simulink model "SST_5"  (R2022b)
settings: Solver=VariableStepAuto  StartTime=0.0  StopTime=1.0  RelTol=1e-3
libraries: spsSeriesRLCBranchLib x13, spsIGBTDiodeLib x10, spsMosfetLib x6, slpidlib x5, spsCurrentMeasurementLib x4, spsDiodeLib x4, spsThreePhaseVIMeasurementLib x3, spsAlphaBetaZerotodq0Lib x2, spsThreePhaseSeriesRLCBranchLib x2, spsVoltageMeasurementLib x2, spsLinearTransformerLib x1, spsGroundLib x1
settings Model: Creator=DR. AGBARAJI  LastModifiedBy=DR. AGBARAJI

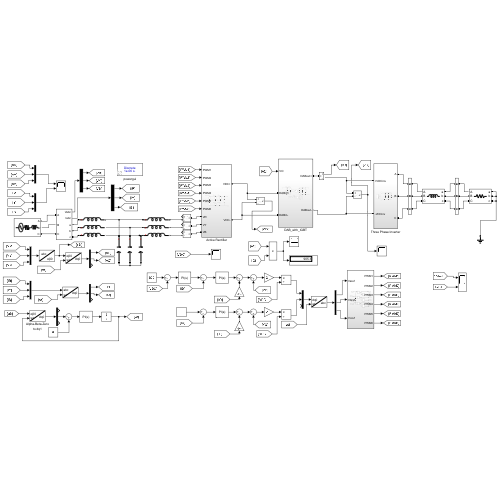
[thumbnail: Simulink's stored preview of the top-level diagram]
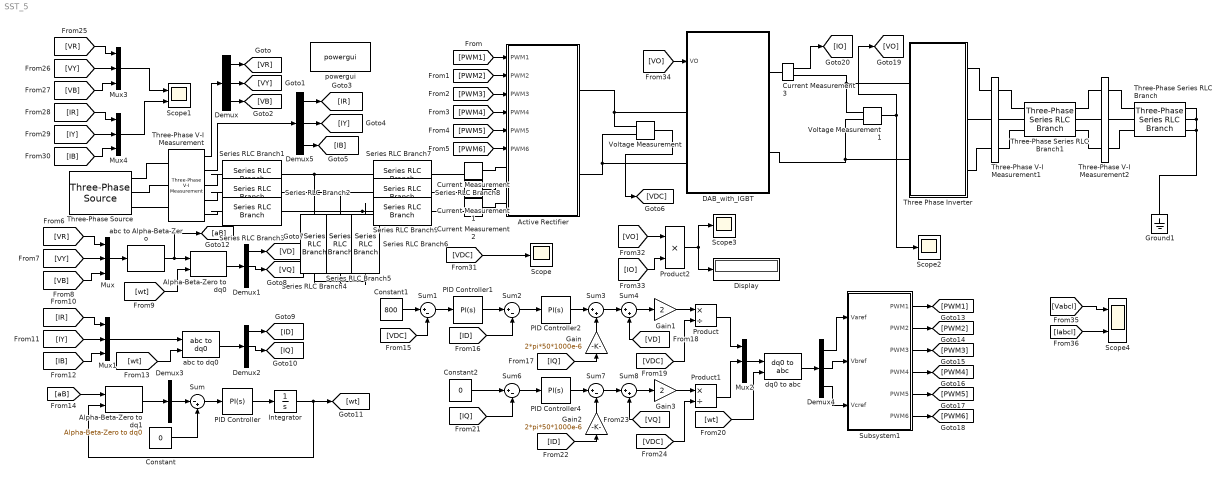
== system SST_5 ==
  Active Rectifier : Subsystem
  Alpha-Beta-Zero to dq0 : spsAlphaBetaZerotodq0Lib/Alpha-Beta-Zero to dq0  Alignment=90 degrees behind phase A axis
  Alpha-Beta-Zero to dq1 : spsAlphaBetaZerotodq0Lib/Alpha-Beta-Zero to dq0  Alignment=90 degrees behind phase A axis
  Constant : Constant  Value=0
  Constant1 : Constant  Value=800
  Constant2 : Constant  Value=0
  Current Measurement{,1..3} (4 alike) : spsCurrentMeasurementLib/Current Measurement  PhasorSimulation=off  OutputType=Complex  PSBequivalent=0
  DAB_with_IGBT : Subsystem
  Demux{,1..5} (6 alike) : Demux  Outputs=3
  Display : Display
  Gain : Gain  Gain=2*pi*50*1000e-6
  Gain1 : Gain  Gain=2
  Gain2 : Gain  Gain=2*pi*50*1000e-6
  Gain3 : Gain  Gain=2
  Ground1 : spsGroundLib/Ground  LConnTagsString=a
  Integrator : Integrator
  Mux{,1..4} (5 alike) : Mux  Inputs=3
  PID Controller : slpidlib/PID Controller  Controller=PI  Form=Parallel  TimeDomain=Continuous-time  UseExternalTs=off  SampleTime=-1  IntegratorMethod=Forward Euler  FilterMethod=Forward Euler  ControllerParametersSource=internal  P=10  I=50000  UseKiTs=off  D=0  N=100  UseFilter=on  TunerSelectOption=Transfer Function Based (PID Tuner App)  InitialConditionSource=internal  InitialConditionForIntegrator=0  InitialConditionForFilter=0  DifferentiatorICPrevScaledInput=0  ExternalReset=none  TrackingMode=off  Kt=1  LimitOutput=off  SatLimitsSource=internal  UpperSaturationLimit=inf  LowerSaturationLimit=-inf  LinearizeAsGain=on  AntiWindupMode=none  Kb=1  LimitIntegrator=off  UpperIntegratorSaturationLimit=inf  LowerIntegratorSaturationLimit=-inf  POutMin=[]  POutMax=[]  IOutMin=[]  IOutMax=[]  DOutMin=[]  DOutMax=[]  NOutMin=[]  NOutMax=[]  SumOutMin=[]  SumOutMax=[]  SaturationOutMin=[]  SaturationOutMax=[]  PParamMin=[]  PParamMax=[]  IParamMin=[]  IParamMax=[]  DParamMin=[]  DParamMax=[]  NParamMin=[]  NParamMax=[]  KbParamMin=[]  KbParamMax=[]  KtParamMin=[]  KtParamMax=[]  KbOutMin=[]  KbOutMax=[]  KtOutMin=[]  KtOutMax=[]  IntegratorOutMin=[]  IntegratorOutMax=[]  FilterOutMin=[]  FilterOutMax=[]  SumI1OutMin=[]  SumI1OutMax=[]  SumI2OutMin=[]  SumI2OutMax=[]  SumI3OutMin=[]  SumI3OutMax=[]  SumI4OutMin=[]  SumI4OutMax=[]  SumDOutMin=[]  SumDOutMax=[]  DifferentiatorOutMin=[]  DifferentiatorOutMax=[]  FilterDiffOutCoefMin=[]  FilterDiffOutCoefMax=[]  ReciprocalOutMin=[]  ReciprocalOutMax=[]  SumDenOutMin=[]  SumDenOutMax=[]  SumNumOutMin=[]  SumNumOutMax=[]  DivideOutMin=[]  DivideOutMax=[]  UdiffTsProdOutMin=[]  UdiffTsProdOutMax=[]  NTsProdOutMin=[]  NTsProdOutMax=[]  UintegralTsProdOutMin=[]  UintegralTsProdOutMax=[]  UngainTsProdOutMin=[]  UngainTsProdOutMax=[]  ClampingZeroOutDataTypeStr=Inherit: Inherit via back propagation  ClampingZeroOutMin=[]  ClampingZeroOutMax=[]  FilterDenConstantOutDataTypeStr=Inherit: Inherit via back propagation  FilterDenConstantOutMin=[]  FilterDenConstantOutMax=[]  PCopyOutDataTypeStr=Inherit: Inherit via back propagation  PCopyOutMin=[]  PCopyOutMax=[]  NCopyOutDataTypeStr=Inherit: Inherit via back propagation  NCopyOutMin=[]  NCopyOutMax=[]  IntegratorContinuousStateAttributes=''  IntegratorStateMustResolveToSignalObject=off  IntegratorRTWStateStorageClass=Auto  FilterContinuousStateAttributes=''  FilterStateMustResolveToSignalObject=off  FilterRTWStateStorageClass=Auto  ParallelPVariant=InternalParameters  IdealPVariant=Disabled  IVariant=InternalParameters  DVariant=Disabled  IntegratorVariant=Continuous  SatVariant=Disabled  AWVariant=Passthrough  PCopyVariant=Disabled  TRVariant=Disabled  FdbkBlocksVariant=Forward  IdealPFdbkVariant=Disabled  SatFdbkVariant=Disabled  DerivativeFilterVariant=Disabled  NVariant=Disabled  NCopyVariant=Disabled_SignalSpec  FilterICVariant=Disabled  IntegratorICVariant=InternalICs  ExternalResetVariant=Disabled  TRSumVariant=Passthrough  SumFdbkVariant=Disabled  SumVariant=Sum_PI  TsampFilterVariant=InternalTs  TsampNgainVariant=Passthrough  TsampIntegralVariant=Passthrough  ExternalSaturationOutDataTypeStr=Inherit: Same as second input
  PID Controller1 : slpidlib/PID Controller  Controller=PI  Form=Parallel  TimeDomain=Continuous-time  UseExternalTs=off  SampleTime=-1  IntegratorMethod=Forward Euler  FilterMethod=Forward Euler  ControllerParametersSource=internal  P=0.5  I=200  UseKiTs=off  D=0  N=100  UseFilter=on  TunerSelectOption=Transfer Function Based (PID Tuner App)  InitialConditionSource=internal  InitialConditionForIntegrator=0  InitialConditionForFilter=0  DifferentiatorICPrevScaledInput=0  ExternalReset=none  TrackingMode=off  Kt=1  LimitOutput=off  SatLimitsSource=internal  UpperSaturationLimit=inf  LowerSaturationLimit=-inf  LinearizeAsGain=on  AntiWindupMode=none  Kb=1  LimitIntegrator=off  UpperIntegratorSaturationLimit=inf  LowerIntegratorSaturationLimit=-inf  POutMin=[]  POutMax=[]  IOutMin=[]  IOutMax=[]  DOutMin=[]  DOutMax=[]  NOutMin=[]  NOutMax=[]  SumOutMin=[]  SumOutMax=[]  SaturationOutMin=[]  SaturationOutMax=[]  PParamMin=[]  PParamMax=[]  IParamMin=[]  IParamMax=[]  DParamMin=[]  DParamMax=[]  NParamMin=[]  NParamMax=[]  KbParamMin=[]  KbParamMax=[]  KtParamMin=[]  KtParamMax=[]  KbOutMin=[]  KbOutMax=[]  KtOutMin=[]  KtOutMax=[]  IntegratorOutMin=[]  IntegratorOutMax=[]  FilterOutMin=[]  FilterOutMax=[]  SumI1OutMin=[]  SumI1OutMax=[]  SumI2OutMin=[]  SumI2OutMax=[]  SumI3OutMin=[]  SumI3OutMax=[]  SumI4OutMin=[]  SumI4OutMax=[]  SumDOutMin=[]  SumDOutMax=[]  DifferentiatorOutMin=[]  DifferentiatorOutMax=[]  FilterDiffOutCoefMin=[]  FilterDiffOutCoefMax=[]  ReciprocalOutMin=[]  ReciprocalOutMax=[]  SumDenOutMin=[]  SumDenOutMax=[]  SumNumOutMin=[]  SumNumOutMax=[]  DivideOutMin=[]  DivideOutMax=[]  UdiffTsProdOutMin=[]  UdiffTsProdOutMax=[]  NTsProdOutMin=[]  NTsProdOutMax=[]  UintegralTsProdOutMin=[]  UintegralTsProdOutMax=[]  UngainTsProdOutMin=[]  UngainTsProdOutMax=[]  ClampingZeroOutDataTypeStr=Inherit: Inherit via back propagation  ClampingZeroOutMin=[]  ClampingZeroOutMax=[]  FilterDenConstantOutDataTypeStr=Inherit: Inherit via back propagation  FilterDenConstantOutMin=[]  FilterDenConstantOutMax=[]  PCopyOutDataTypeStr=Inherit: Inherit via back propagation  PCopyOutMin=[]  PCopyOutMax=[]  NCopyOutDataTypeStr=Inherit: Inherit via back propagation  NCopyOutMin=[]  NCopyOutMax=[]  IntegratorContinuousStateAttributes=''  IntegratorStateMustResolveToSignalObject=off  IntegratorRTWStateStorageClass=Auto  FilterContinuousStateAttributes=''  FilterStateMustResolveToSignalObject=off  FilterRTWStateStorageClass=Auto  ParallelPVariant=InternalParameters  IdealPVariant=Disabled  IVariant=InternalParameters  DVariant=Disabled  IntegratorVariant=Continuous  SatVariant=Disabled  AWVariant=Passthrough  PCopyVariant=Disabled  TRVariant=Disabled  FdbkBlocksVariant=Forward  IdealPFdbkVariant=Disabled  SatFdbkVariant=Disabled  DerivativeFilterVariant=Disabled  NVariant=Disabled  NCopyVariant=Disabled_SignalSpec  FilterICVariant=Disabled  IntegratorICVariant=InternalICs  ExternalResetVariant=Disabled  TRSumVariant=Passthrough  SumFdbkVariant=Disabled  SumVariant=Sum_PI  TsampFilterVariant=InternalTs  TsampNgainVariant=Passthrough  TsampIntegralVariant=Passthrough  ExternalSaturationOutDataTypeStr=Inherit: Same as second input
  PID Controller2 : slpidlib/PID Controller  Controller=PI  Form=Parallel  TimeDomain=Continuous-time  UseExternalTs=off  SampleTime=-1  IntegratorMethod=Forward Euler  FilterMethod=Forward Euler  ControllerParametersSource=internal  P=25  I=500  UseKiTs=off  D=0  N=100  UseFilter=on  TunerSelectOption=Transfer Function Based (PID Tuner App)  InitialConditionSource=internal  InitialConditionForIntegrator=0  InitialConditionForFilter=0  DifferentiatorICPrevScaledInput=0  ExternalReset=none  TrackingMode=off  Kt=1  LimitOutput=off  SatLimitsSource=internal  UpperSaturationLimit=inf  LowerSaturationLimit=-inf  LinearizeAsGain=on  AntiWindupMode=none  Kb=1  LimitIntegrator=off  UpperIntegratorSaturationLimit=inf  LowerIntegratorSaturationLimit=-inf  POutMin=[]  POutMax=[]  IOutMin=[]  IOutMax=[]  DOutMin=[]  DOutMax=[]  NOutMin=[]  NOutMax=[]  SumOutMin=[]  SumOutMax=[]  SaturationOutMin=[]  SaturationOutMax=[]  PParamMin=[]  PParamMax=[]  IParamMin=[]  IParamMax=[]  DParamMin=[]  DParamMax=[]  NParamMin=[]  NParamMax=[]  KbParamMin=[]  KbParamMax=[]  KtParamMin=[]  KtParamMax=[]  KbOutMin=[]  KbOutMax=[]  KtOutMin=[]  KtOutMax=[]  IntegratorOutMin=[]  IntegratorOutMax=[]  FilterOutMin=[]  FilterOutMax=[]  SumI1OutMin=[]  SumI1OutMax=[]  SumI2OutMin=[]  SumI2OutMax=[]  SumI3OutMin=[]  SumI3OutMax=[]  SumI4OutMin=[]  SumI4OutMax=[]  SumDOutMin=[]  SumDOutMax=[]  DifferentiatorOutMin=[]  DifferentiatorOutMax=[]  FilterDiffOutCoefMin=[]  FilterDiffOutCoefMax=[]  ReciprocalOutMin=[]  ReciprocalOutMax=[]  SumDenOutMin=[]  SumDenOutMax=[]  SumNumOutMin=[]  SumNumOutMax=[]  DivideOutMin=[]  DivideOutMax=[]  UdiffTsProdOutMin=[]  UdiffTsProdOutMax=[]  NTsProdOutMin=[]  NTsProdOutMax=[]  UintegralTsProdOutMin=[]  UintegralTsProdOutMax=[]  UngainTsProdOutMin=[]  UngainTsProdOutMax=[]  ClampingZeroOutDataTypeStr=Inherit: Inherit via back propagation  ClampingZeroOutMin=[]  ClampingZeroOutMax=[]  FilterDenConstantOutDataTypeStr=Inherit: Inherit via back propagation  FilterDenConstantOutMin=[]  FilterDenConstantOutMax=[]  PCopyOutDataTypeStr=Inherit: Inherit via back propagation  PCopyOutMin=[]  PCopyOutMax=[]  NCopyOutDataTypeStr=Inherit: Inherit via back propagation  NCopyOutMin=[]  NCopyOutMax=[]  IntegratorContinuousStateAttributes=''  IntegratorStateMustResolveToSignalObject=off  IntegratorRTWStateStorageClass=Auto  FilterContinuousStateAttributes=''  FilterStateMustResolveToSignalObject=off  FilterRTWStateStorageClass=Auto  ParallelPVariant=InternalParameters  IdealPVariant=Disabled  IVariant=InternalParameters  DVariant=Disabled  IntegratorVariant=Continuous  SatVariant=Disabled  AWVariant=Passthrough  PCopyVariant=Disabled  TRVariant=Disabled  FdbkBlocksVariant=Forward  IdealPFdbkVariant=Disabled  SatFdbkVariant=Disabled  DerivativeFilterVariant=Disabled  NVariant=Disabled  NCopyVariant=Disabled_SignalSpec  FilterICVariant=Disabled  IntegratorICVariant=InternalICs  ExternalResetVariant=Disabled  TRSumVariant=Passthrough  SumFdbkVariant=Disabled  SumVariant=Sum_PI  TsampFilterVariant=InternalTs  TsampNgainVariant=Passthrough  TsampIntegralVariant=Passthrough  ExternalSaturationOutDataTypeStr=Inherit: Same as second input
  PID Controller4 : slpidlib/PID Controller  Controller=PI  Form=Parallel  TimeDomain=Continuous-time  UseExternalTs=off  SampleTime=-1  IntegratorMethod=Forward Euler  FilterMethod=Forward Euler  ControllerParametersSource=internal  P=25  I=500  UseKiTs=off  D=0  N=100  UseFilter=on  TunerSelectOption=Transfer Function Based (PID Tuner App)  InitialConditionSource=internal  InitialConditionForIntegrator=0  InitialConditionForFilter=0  DifferentiatorICPrevScaledInput=0  ExternalReset=none  TrackingMode=off  Kt=1  LimitOutput=off  SatLimitsSource=internal  UpperSaturationLimit=inf  LowerSaturationLimit=-inf  LinearizeAsGain=on  AntiWindupMode=none  Kb=1  LimitIntegrator=off  UpperIntegratorSaturationLimit=inf  LowerIntegratorSaturationLimit=-inf  POutMin=[]  POutMax=[]  IOutMin=[]  IOutMax=[]  DOutMin=[]  DOutMax=[]  NOutMin=[]  NOutMax=[]  SumOutMin=[]  SumOutMax=[]  SaturationOutMin=[]  SaturationOutMax=[]  PParamMin=[]  PParamMax=[]  IParamMin=[]  IParamMax=[]  DParamMin=[]  DParamMax=[]  NParamMin=[]  NParamMax=[]  KbParamMin=[]  KbParamMax=[]  KtParamMin=[]  KtParamMax=[]  KbOutMin=[]  KbOutMax=[]  KtOutMin=[]  KtOutMax=[]  IntegratorOutMin=[]  IntegratorOutMax=[]  FilterOutMin=[]  FilterOutMax=[]  SumI1OutMin=[]  SumI1OutMax=[]  SumI2OutMin=[]  SumI2OutMax=[]  SumI3OutMin=[]  SumI3OutMax=[]  SumI4OutMin=[]  SumI4OutMax=[]  SumDOutMin=[]  SumDOutMax=[]  DifferentiatorOutMin=[]  DifferentiatorOutMax=[]  FilterDiffOutCoefMin=[]  FilterDiffOutCoefMax=[]  ReciprocalOutMin=[]  ReciprocalOutMax=[]  SumDenOutMin=[]  SumDenOutMax=[]  SumNumOutMin=[]  SumNumOutMax=[]  DivideOutMin=[]  DivideOutMax=[]  UdiffTsProdOutMin=[]  UdiffTsProdOutMax=[]  NTsProdOutMin=[]  NTsProdOutMax=[]  UintegralTsProdOutMin=[]  UintegralTsProdOutMax=[]  UngainTsProdOutMin=[]  UngainTsProdOutMax=[]  ClampingZeroOutDataTypeStr=Inherit: Inherit via back propagation  ClampingZeroOutMin=[]  ClampingZeroOutMax=[]  FilterDenConstantOutDataTypeStr=Inherit: Inherit via back propagation  FilterDenConstantOutMin=[]  FilterDenConstantOutMax=[]  PCopyOutDataTypeStr=Inherit: Inherit via back propagation  PCopyOutMin=[]  PCopyOutMax=[]  NCopyOutDataTypeStr=Inherit: Inherit via back propagation  NCopyOutMin=[]  NCopyOutMax=[]  IntegratorContinuousStateAttributes=''  IntegratorStateMustResolveToSignalObject=off  IntegratorRTWStateStorageClass=Auto  FilterContinuousStateAttributes=''  FilterStateMustResolveToSignalObject=off  FilterRTWStateStorageClass=Auto  ParallelPVariant=InternalParameters  IdealPVariant=Disabled  IVariant=InternalParameters  DVariant=Disabled  IntegratorVariant=Continuous  SatVariant=Disabled  AWVariant=Passthrough  PCopyVariant=Disabled  TRVariant=Disabled  FdbkBlocksVariant=Forward  IdealPFdbkVariant=Disabled  SatFdbkVariant=Disabled  DerivativeFilterVariant=Disabled  NVariant=Disabled  NCopyVariant=Disabled_SignalSpec  FilterICVariant=Disabled  IntegratorICVariant=InternalICs  ExternalResetVariant=Disabled  TRSumVariant=Passthrough  SumFdbkVariant=Disabled  SumVariant=Sum_PI  TsampFilterVariant=InternalTs  TsampNgainVariant=Passthrough  TsampIntegralVariant=Passthrough  ExternalSaturationOutDataTypeStr=Inherit: Same as second input
  Product : Product  Inputs=*/
  Product1 : Product  Inputs=*/
  Product2 : Product
  Scope : Scope
  Scope1 : Scope  NumInputPorts=2
  Scope2 : Scope
  Scope3 : Scope
  Scope4 : Scope  NumInputPorts=2
  Series RLC Branch{1..3,7..9} (6 alike) : spsSeriesRLCBranchLib/Series RLC Branch  LConnTagsString=__new0  RConnTagsString=__new0  BranchType=L  Resistance=1  Inductance=500e-6  SetiL0=off  InitialCurrent=0  Capacitance=1e-6  Setx0=off  InitialVoltage=0  Measurements=None
  Series RLC Branch4 : spsSeriesRLCBranchLib/Series RLC Branch  LConnTagsString=__new0  RConnTagsString=__new0  BranchType=C  Resistance=1  Inductance=1e-3  SetiL0=off  InitialCurrent=0  Capacitance=100e-6  Setx0=off  InitialVoltage=0  Measurements=None
  Series RLC Branch5 : spsSeriesRLCBranchLib/Series RLC Branch  LConnTagsString=__new0  RConnTagsString=__new0  BranchType=C  Resistance=1  Inductance=1e-3  SetiL0=off  InitialCurrent=0  Capacitance=100e-6  Setx0=off  InitialVoltage=0  Measurements=None
  Series RLC Branch6 : spsSeriesRLCBranchLib/Series RLC Branch  LConnTagsString=__new0  RConnTagsString=__new0  BranchType=C  Resistance=1  Inductance=1e-3  SetiL0=off  InitialCurrent=0  Capacitance=100e-6  Setx0=off  InitialVoltage=0  Measurements=None
  Subsystem1 : Subsystem
  Sum : Sum  Inputs=|-+
  Sum{1..2,6..7} (4 alike) : Sum  Inputs=|+-
  Sum3 : Sum  Inputs=|++
  Sum4 : Sum  Inputs=|++
  Sum8 : Sum  Inputs=|++
  Three Phase Inverter : Subsystem
  Three-Phase Series RLC Branch : spsThreePhaseSeriesRLCBranchLib/Three-Phase Series RLC Branch  LConnTagsString=A|B|C  RConnTagsString=A|B|C  BranchType=R  Resistance=80  Inductance=1e-3  Capacitance=1e-6  Measurements=None
  Three-Phase Series RLC Branch1 : spsThreePhaseSeriesRLCBranchLib/Three-Phase Series RLC Branch  LConnTagsString=A|B|C  RConnTagsString=A|B|C  BranchType=L  Resistance=1  Inductance=9e-3  Capacitance=1e-6  Measurements=None
  Three-Phase V-I Measurement : spsThreePhaseVIMeasurementLib/Three-Phase V-I Measurement  VoltageMeasurement=phase-to-phase  SetLabelV=off  LabelV=Vabc  Vpu=off  VpuLL=off  CurrentMeasurement=yes  SetLabelI=off  LabelI=Iabc  Ipu=off  Pbase=100e6  Vbase=500e3  OutputType=Complex  PhasorSimulation=off  PSBequivalent=0
  Three-Phase V-I Measurement1 : spsThreePhaseVIMeasurementLib/Three-Phase V-I Measurement  VoltageMeasurement=phase-to-ground  SetLabelV=on  LabelV=Vabc  Vpu=off  VpuLL=off  CurrentMeasurement=yes  SetLabelI=on  LabelI=Iabc  Ipu=off  Pbase=100e6  Vbase=500e3  OutputType=Complex  PhasorSimulation=off  PSBequivalent=0
  Three-Phase V-I Measurement2 : spsThreePhaseVIMeasurementLib/Three-Phase V-I Measurement  VoltageMeasurement=phase-to-ground  SetLabelV=on  LabelV=Vabcl  Vpu=off  VpuLL=off  CurrentMeasurement=yes  SetLabelI=on  LabelI=Iabcl  Ipu=off  Pbase=100e6  Vbase=500e3  OutputType=Complex  PhasorSimulation=off  PSBequivalent=0
  Three-Phase Source : spsThreePhaseSourceLib/Three-Phase Source  InternalConnection=Y  VoltagePhases=off  Voltage=415  PhaseAngle=0  Voltage_phases=[25e3 25e3 25e3]/sqrt(3)  PhaseAngles_phases=[0 -120 +120]  Frequency=50  NonIdealSource=on  SpecifyImpedance=off  Resistance=0.8929e-3  Inductance=16.58e-6  ShortCircuitLevel=100e6  BaseVoltage=415  XRratio=7  BusType=swing  Pref=10e3  Qref=0  Prefabc=[10e3, 10e3, 10e3]  Qrefabc=[0, 0, 0]  Qmin=-inf  Qmax=inf
  Voltage Measurement : spsVoltageMeasurementLib/Voltage Measurement  PhasorSimulation=off  OutputType=Complex  PSBequivalent=0
  Voltage Measurement1 : spsVoltageMeasurementLib/Voltage Measurement  PhasorSimulation=off  OutputType=Complex  PSBequivalent=0
  abc to Alpha-Beta-Zero : spsabctoAlphaBetaZeroLib/abc to Alpha-Beta-Zero
  abc to dq0 : spsabctodq0Lib/abc to dq0  Alignment=90 degrees behind phase A axis
  dq0 to abc : spsdq0toabcLib/dq0 to abc  Alignment=90 degrees behind phase A axis
  powergui : sps_lib/powergui  Priority=1  SimulationMode=Discrete  SampleTime=1e-6  frequency=60  Iterations=50  frequencyindice=50  Pbase=100e6  ErrMax=1e-4  UnitsV=kV  UnitsW=MW  buscounter=0  FunctionMessages=off  echomessages=off  EnableUseOfTLC=off  CurrentSourceSwitches=off  DisableSnubberDevices=off  DisableRonSwitches=off  DisableVfSwitches=off  DisplayEquations=off  AutomaticDiscreteSolvers=off  SolverType=Tustin/Backward Euler (TBE)  Interpol=off  ExternalGateDelay=off  methode=off  Ts=100  x0status=blocks  SPID=on  SwTol=0  HookPort=off  NonlinearTolerance=1e-4  nMaxIteration=100  ContinueOnMaxIteration=off  RestoreLinks=warning  ResistiveCurrentMeasurement=off  Frange=[0:2:500]  Ylog=off  Xlog=on  ShowGrid=off  save=off  variable=ZData  structure=0  ZoomFFT=off  StartTime=0.0  cycles=1  DisplayStyle=1  fundamental=60  FreqAxis=off  MaxFrequency=1000  frequencyindicesteady=1  RmsSteady=1  display=off
  wires:
  Demux3/2 -> Sum/1
  [wt] -> abc to dq0/2
  Demux1/2 -> [VQ]
  [wt] -> Alpha-Beta-Zero to dq0/2
  Demux1/1 -> [VD]
  Mux/1 -> abc to Alpha-Beta-Zero/1
  [VY] -> Mux/2
  [VR] -> Mux/1
  abc to Alpha-Beta-Zero/1 -> [aB], Alpha-Beta-Zero to dq0/1
  [IR] -> Mux1/1
  Demux2/2 -> [IQ]
  [PWM5] -> Active Rectifier/5(PWM5)
  [PWM6] -> Active Rectifier/6(PWM6)
  Voltage Measurement/1 -> [VDC]
  [PWM4] -> Active Rectifier/4(PWM4)
  [PWM1] -> Active Rectifier/1(PWM1)
  [PWM3] -> Active Rectifier/3(PWM3)
  Demux4/3 -> Subsystem1/3(Vcref)
  [VY] -> Mux3/2
  Sum3/1 -> Sum4/1
  Alpha-Beta-Zero to dq0/1 -> Demux1/1
  Sum1/1 -> PID Controller1/1
  Alpha-Beta-Zero to dq1/1 -> Demux3/1
  [VDC] -> Scope/1
  PID Controller4/1 -> Sum7/1
  Mux2/1 -> dq0 to abc/1
  [VR] -> Mux3/1
  Three-Phase V-I Measurement/1 -> Demux/1
  Mux3/1 -> Scope1/1
  [IR] -> Mux4/1
  [ID] -> Gain2/1
  [VB] -> Mux3/3
  Constant2/1 -> Sum6/1
  Demux/3 -> [VB]
  Demux/1 -> [VR]
  PID Controller1/1 -> Sum2/1
  [wt] -> dq0 to abc/2
  [IB] -> Mux1/3
  Integrator/1 -> [wt], Alpha-Beta-Zero to dq1/2
  Subsystem1/1(PWM1) -> [PWM1]
  Subsystem1/4(PWM4) -> [PWM4]
  Subsystem1/5(PWM5) -> [PWM5]
  Gain2/1 -> Sum7/2
  Subsystem1/6(PWM6) -> [PWM6]
  Sum2/1 -> PID Controller2/1
  dq0 to abc/1 -> Demux4/1
  Mux4/1 -> Scope1/2
  [IQ] -> Sum6/2
  PID Controller2/1 -> Sum3/1
  Demux/2 -> [VY]
  Gain1/1 -> Product/1
  [IB] -> Mux4/3
  Demux4/2 -> Subsystem1/2(Vbref)
  Product/1 -> Mux2/1
  [IY] -> Mux1/2
  [IY] -> Mux4/2
  Mux1/1 -> abc to dq0/1
  Sum8/1 -> Gain3/1
  abc to dq0/1 -> Demux2/1
  Sum7/1 -> Sum8/1
  [VDC] -> Product1/2
  Subsystem1/3(PWM3) -> [PWM3]
  [VDC] -> Product/2
  [VQ] -> Sum8/2
  Sum4/1 -> Gain1/1
  Sum6/1 -> PID Controller4/1
  [IQ] -> Gain/1
  Demux4/1 -> Subsystem1/1(Varef)
  Gain3/1 -> Product1/1
  Gain/1 -> Sum3/2
  Demux2/1 -> [ID]
  [PWM2] -> Active Rectifier/2(PWM2)
  PID Controller/1 -> Integrator/1
  Sum/1 -> PID Controller/1
  [ID] -> Sum2/2
  Constant/1 -> Sum/2
  Subsystem1/2(PWM2) -> [PWM2]
  [VB] -> Mux/3
  [VD] -> Sum4/2
  Product1/1 -> Mux2/2
  Constant1/1 -> Sum1/1
  [VDC] -> Sum1/2
  [aB] -> Alpha-Beta-Zero to dq1/1
  Voltage Measurement1/1 -> Scope2/1, [VO]
  Current Measurement3/1 -> [IO]
  [VO] -> Product2/1
  Product2/1 -> Display/1, Scope3/1
  [VO] -> DAB_with_IGBT/1(VO)
  [IO] -> Product2/2
  [Vabcl] -> Scope4/1
  [Iabcl] -> Scope4/2
  Demux5/3 -> [IB]
  Demux5/2 -> [IY]
  Demux5/1 -> [IR]
  Three-Phase V-I Measurement/2 -> Demux5/1
  connections:
  Voltage Measurement/LConn2 -- Active Rectifier/RConn2 -- DAB_with_IGBT/LConn2
  Series RLC Branch7/LConn1 -- Series RLC Branch4/LConn1 -- Series RLC Branch1/RConn1
  Series RLC Branch9/LConn1 -- Series RLC Branch6/LConn1 -- Series RLC Branch3/RConn1
  Series RLC Branch8/LConn1 -- Series RLC Branch5/LConn1 -- Series RLC Branch2/RConn1
  Series RLC Branch5/RConn1 -- Series RLC Branch6/RConn1 -- Series RLC Branch4/RConn1
  Voltage Measurement/LConn1 -- Active Rectifier/RConn1 -- DAB_with_IGBT/LConn1
  Current Measurement1/RConn1 -- Series RLC Branch8/RConn1
  Series RLC Branch1/LConn1 -- Three-Phase V-I Measurement/RConn1
  Current Measurement2/RConn1 -- Series RLC Branch9/RConn1
  Three-Phase V-I Measurement/LConn1 -- Three-Phase Source/RConn1
  Active Rectifier/LConn3 -- Current Measurement2/LConn1
  Three-Phase Source/RConn3 -- Three-Phase V-I Measurement/LConn3
  Three-Phase V-I Measurement/LConn2 -- Three-Phase Source/RConn2
  Active Rectifier/LConn2 -- Current Measurement1/LConn1
  Active Rectifier/LConn1 -- Current Measurement/LConn1
  Series RLC Branch2/LConn1 -- Three-Phase V-I Measurement/RConn2
  Current Measurement/RConn1 -- Series RLC Branch7/RConn1
  Series RLC Branch3/LConn1 -- Three-Phase V-I Measurement/RConn3
  Current Measurement3/RConn1 -- Three Phase Inverter/LConn1 -- Voltage Measurement1/LConn1
  Three Phase Inverter/LConn2 -- DAB_with_IGBT/RConn2 -- Voltage Measurement1/LConn2
  Current Measurement3/LConn1 -- DAB_with_IGBT/RConn1
  Three-Phase Series RLC Branch/RConn3 -- Ground1/LConn1 -- Three-Phase Series RLC Branch/RConn2 -- Three-Phase Series RLC Branch/RConn1
  Three-Phase Series RLC Branch/LConn1 -- Three-Phase V-I Measurement2/RConn1
  Three-Phase V-I Measurement1/RConn2 -- Three-Phase Series RLC Branch1/LConn2
  Three-Phase V-I Measurement2/RConn3 -- Three-Phase Series RLC Branch/LConn3
  Three-Phase V-I Measurement1/RConn1 -- Three-Phase Series RLC Branch1/LConn1
  Three-Phase V-I Measurement1/LConn3 -- Three Phase Inverter/RConn3
  Three-Phase V-I Measurement1/LConn1 -- Three Phase Inverter/RConn1
  Three-Phase V-I Measurement1/RConn3 -- Three-Phase Series RLC Branch1/LConn3
  Three-Phase Series RLC Branch1/RConn2 -- Three-Phase V-I Measurement2/LConn2
  Three-Phase V-I Measurement1/LConn2 -- Three Phase Inverter/RConn2
  Three-Phase Series RLC Branch1/RConn3 -- Three-Phase V-I Measurement2/LConn3
  Three-Phase Series RLC Branch1/RConn1 -- Three-Phase V-I Measurement2/LConn1
  Three-Phase V-I Measurement2/RConn2 -- Three-Phase Series RLC Branch/LConn2

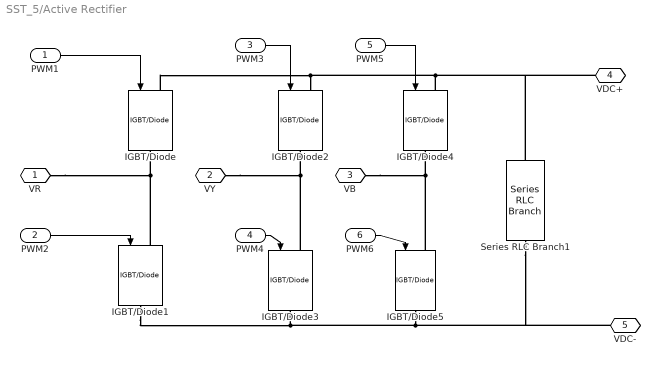
== system SST_5/Active Rectifier ==
  PWM1 : Inport
  PWM2 : Inport  Port=2
  PWM3 : Inport  Port=3
  PWM4 : Inport  Port=4
  PWM5 : Inport  Port=5
  PWM6 : Inport  Port=6
  IGBT/Diode{,1..5} (6 alike) : spsIGBTDiodeLib/IGBT//Diode  Ron=1e-3  Rs=1e5  Cs=inf  Measurements=off
  Series RLC Branch1 : spsSeriesRLCBranchLib/Series RLC Branch  LConnTagsString=__new0  RConnTagsString=__new0  BranchType=RC  Resistance=1e-3  Inductance=1e-3  SetiL0=off  InitialCurrent=0  Capacitance=5600e-6  Setx0=off  InitialVoltage=0  Measurements=None
  VR : PMIOPort  Side=Left
  VY : PMIOPort  Port=2  Side=Left
  VB : PMIOPort  Port=3  Side=Left
  VDC+ : PMIOPort  Port=4  Side=Right
  VDC- : PMIOPort  Port=5  Side=Right
  wires:
  PWM3/1 -> IGBT/Diode2/1
  PWM4/1 -> IGBT/Diode3/1
  PWM6/1 -> IGBT/Diode5/1
  PWM5/1 -> IGBT/Diode4/1
  PWM1/1 -> IGBT/Diode/1
  PWM2/1 -> IGBT/Diode1/1
  connections:
  IGBT/Diode5/RConn1 -- VDC-/RConn1 -- Series RLC Branch1/RConn1 -- IGBT/Diode1/RConn1 -- IGBT/Diode3/RConn1
  IGBT/Diode5/LConn1 -- VB/RConn1 -- IGBT/Diode4/RConn1
  IGBT/Diode4/LConn1 -- VDC+/RConn1 -- Series RLC Branch1/LConn1 -- IGBT/Diode/LConn1 -- IGBT/Diode2/LConn1
  IGBT/Diode1/LConn1 -- VR/RConn1 -- IGBT/Diode/RConn1
  IGBT/Diode3/LConn1 -- VY/RConn1 -- IGBT/Diode2/RConn1

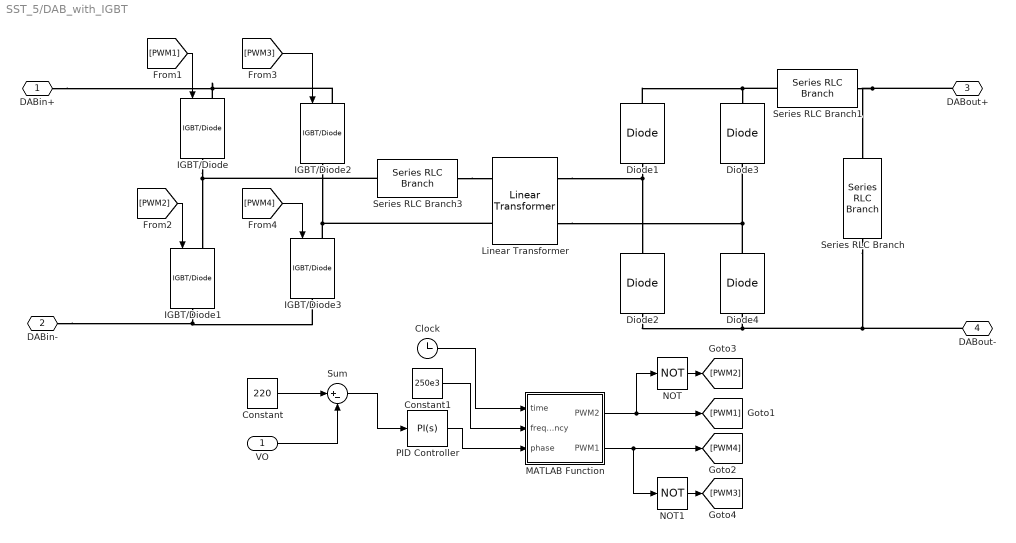
== system SST_5/DAB_with_IGBT ==
  VO : Inport
  Clock : Clock
  Constant : Constant  Value=220
  Constant1 : Constant  Value=250e3
  Diode{1..4} (4 alike) : spsDiodeLib/Diode  Ron=0.001  Lon=0  Vf=0.8  IC=0  UseSnubber=0  Rs=500  Cs=250e-9  Measurements=off
  IGBT/Diode{,1..3} (4 alike) : spsIGBTDiodeLib/IGBT//Diode  Ron=1e-3  Rs=1e5  Cs=inf  Measurements=off
  Linear Transformer : spsLinearTransformerLib/Linear Transformer  UNITS=SI  NominalPower=[ 480 250e3 ]  winding1=[600 4e-9 0.5e-9]  winding2=[250 0.5e-9 0.05e-9]  ThreeWindings=off  winding3=[3.15e+05 0.7938 0.084225]  RmLm=[1e6 2800]  Measurements=None  DataType=on
  MATLAB Function : MATLAB Function  TreatAsAtomicUnit=on
  NOT : Logic  Operator=NOT  IconShape=distinctive  AllPortsSameDT=off  OutDataTypeStr=boolean
  NOT1 : Logic  Operator=NOT  IconShape=distinctive  AllPortsSameDT=off  OutDataTypeStr=boolean
  PID Controller : slpidlib/PID Controller  Controller=PI  Form=Parallel  TimeDomain=Continuous-time  UseExternalTs=off  SampleTime=-1  IntegratorMethod=Forward Euler  FilterMethod=Forward Euler  ControllerParametersSource=internal  P=50000  I=5000  UseKiTs=off  D=0  N=100  UseFilter=on  TunerSelectOption=Transfer Function Based (PID Tuner App)  InitialConditionSource=internal  InitialConditionForIntegrator=0  InitialConditionForFilter=0  DifferentiatorICPrevScaledInput=0  ExternalReset=none  TrackingMode=off  Kt=1  LimitOutput=on  SatLimitsSource=internal  UpperSaturationLimit=180  LowerSaturationLimit=-inf  LinearizeAsGain=on  AntiWindupMode=none  Kb=1  LimitIntegrator=off  UpperIntegratorSaturationLimit=inf  LowerIntegratorSaturationLimit=-inf  POutMin=[]  POutMax=[]  IOutMin=[]  IOutMax=[]  DOutMin=[]  DOutMax=[]  NOutMin=[]  NOutMax=[]  SumOutMin=[]  SumOutMax=[]  SaturationOutMin=[]  SaturationOutMax=[]  PParamMin=[]  PParamMax=[]  IParamMin=[]  IParamMax=[]  DParamMin=[]  DParamMax=[]  NParamMin=[]  NParamMax=[]  KbParamMin=[]  KbParamMax=[]  KtParamMin=[]  KtParamMax=[]  KbOutMin=[]  KbOutMax=[]  KtOutMin=[]  KtOutMax=[]  IntegratorOutMin=[]  IntegratorOutMax=[]  FilterOutMin=[]  FilterOutMax=[]  SumI1OutMin=[]  SumI1OutMax=[]  SumI2OutMin=[]  SumI2OutMax=[]  SumI3OutMin=[]  SumI3OutMax=[]  SumI4OutMin=[]  SumI4OutMax=[]  SumDOutMin=[]  SumDOutMax=[]  DifferentiatorOutMin=[]  DifferentiatorOutMax=[]  FilterDiffOutCoefMin=[]  FilterDiffOutCoefMax=[]  ReciprocalOutMin=[]  ReciprocalOutMax=[]  SumDenOutMin=[]  SumDenOutMax=[]  SumNumOutMin=[]  SumNumOutMax=[]  DivideOutMin=[]  DivideOutMax=[]  UdiffTsProdOutMin=[]  UdiffTsProdOutMax=[]  NTsProdOutMin=[]  NTsProdOutMax=[]  UintegralTsProdOutMin=[]  UintegralTsProdOutMax=[]  UngainTsProdOutMin=[]  UngainTsProdOutMax=[]  ClampingZeroOutDataTypeStr=Inherit: Inherit via back propagation  ClampingZeroOutMin=[]  ClampingZeroOutMax=[]  FilterDenConstantOutDataTypeStr=Inherit: Inherit via back propagation  FilterDenConstantOutMin=[]  FilterDenConstantOutMax=[]  PCopyOutDataTypeStr=Inherit: Inherit via back propagation  PCopyOutMin=[]  PCopyOutMax=[]  NCopyOutDataTypeStr=Inherit: Inherit via back propagation  NCopyOutMin=[]  NCopyOutMax=[]  IntegratorContinuousStateAttributes=''  IntegratorStateMustResolveToSignalObject=off  IntegratorRTWStateStorageClass=Auto  FilterContinuousStateAttributes=''  FilterStateMustResolveToSignalObject=off  FilterRTWStateStorageClass=Auto  ParallelPVariant=InternalParameters  IdealPVariant=Disabled  IVariant=InternalParameters  DVariant=Disabled  IntegratorVariant=Continuous  SatVariant=Enabled  AWVariant=Passthrough  PCopyVariant=Disabled  TRVariant=Disabled  FdbkBlocksVariant=Forward  IdealPFdbkVariant=Disabled  SatFdbkVariant=Disabled  DerivativeFilterVariant=Disabled  NVariant=Disabled  NCopyVariant=Disabled_SignalSpec  FilterICVariant=Disabled  IntegratorICVariant=InternalICs  ExternalResetVariant=Disabled  TRSumVariant=Passthrough  SumFdbkVariant=Disabled  SumVariant=Sum_PI  TsampFilterVariant=InternalTs  TsampNgainVariant=Passthrough  TsampIntegralVariant=Passthrough  ExternalSaturationOutDataTypeStr=Inherit: Same as second input
  Series RLC Branch : spsSeriesRLCBranchLib/Series RLC Branch  LConnTagsString=__new0  RConnTagsString=__new0  BranchType=C  Resistance=1  Inductance=1e-3  SetiL0=off  InitialCurrent=0  Capacitance=106e-3  Setx0=off  InitialVoltage=0  Measurements=None
  Series RLC Branch1 : spsSeriesRLCBranchLib/Series RLC Branch  LConnTagsString=__new0  RConnTagsString=__new0  BranchType=L  Resistance=1  Inductance=0.6e-9  SetiL0=off  InitialCurrent=0  Capacitance=1e-6  Setx0=off  InitialVoltage=0  Measurements=None
  Series RLC Branch3 : spsSeriesRLCBranchLib/Series RLC Branch  LConnTagsString=__new0  RConnTagsString=__new0  BranchType=L  Resistance=1  Inductance=0.0006e-6  SetiL0=off  InitialCurrent=0  Capacitance=1e-6  Setx0=off  InitialVoltage=0  Measurements=None
  Sum : Sum  Inputs=|+-
  DABin+ : PMIOPort  Side=Left
  DABin- : PMIOPort  Port=2  Side=Left
  DABout+ : PMIOPort  Port=3  Side=Right
  DABout- : PMIOPort  Port=4  Side=Right
  wires:
  [PWM4] -> IGBT/Diode3/1
  [PWM1] -> IGBT/Diode/1
  PID Controller/1 -> MATLAB Function/3(phase)
  Constant/1 -> Sum/1
  MATLAB Function/2(PWM1) -> NOT1/1, [PWM4]
  NOT/1 -> [PWM2]
  Sum/1 -> PID Controller/1
  [PWM2] -> IGBT/Diode1/1
  VO/1 -> Sum/2
  Constant1/1 -> MATLAB Function/2(frequency)
  NOT1/1 -> [PWM3]
  Clock/1 -> MATLAB Function/1(time)
  MATLAB Function/1(PWM2) -> NOT/1, [PWM1]
  [PWM3] -> IGBT/Diode2/1
  connections:
  Linear Transformer/RConn2 -- Diode3/LConn1 -- Diode4/RConn1
  IGBT/Diode1/RConn1 -- IGBT/Diode3/RConn1 -- DABin-/RConn1
  Diode3/RConn1 -- Series RLC Branch1/LConn1 -- Diode1/RConn1
  IGBT/Diode/RConn1 -- Series RLC Branch3/LConn1 -- IGBT/Diode1/LConn1
  DABout+/RConn1 -- Series RLC Branch1/RConn1 -- Series RLC Branch/LConn1
  Diode1/LConn1 -- Linear Transformer/RConn1 -- Diode2/RConn1
  IGBT/Diode2/RConn1 -- Linear Transformer/LConn2 -- IGBT/Diode3/LConn1
  IGBT/Diode/LConn1 -- DABin+/RConn1 -- IGBT/Diode2/LConn1
  Series RLC Branch3/RConn1 -- Linear Transformer/LConn1
  DABout-/RConn1 -- Series RLC Branch/RConn1 -- Diode2/LConn1 -- Diode4/LConn1

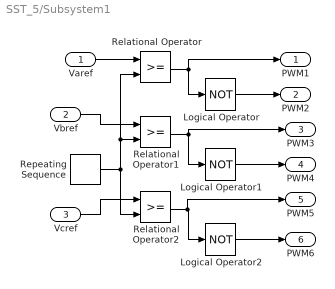
== system SST_5/Subsystem1 ==
  Varef : Inport
  Vbref : Inport  Port=2
  Vcref : Inport  Port=3
  Logical Operator : Logic  Operator=NOT  AllPortsSameDT=off  OutDataTypeStr=boolean
  Logical Operator1 : Logic  Operator=NOT  AllPortsSameDT=off  OutDataTypeStr=boolean
  Logical Operator2 : Logic  Operator=NOT  AllPortsSameDT=off  OutDataTypeStr=boolean
  Relational Operator : RelationalOperator  OutDataTypeStr=boolean  RndMeth=Simplest  InputSameDT=off
  Relational Operator1 : RelationalOperator  OutDataTypeStr=boolean  RndMeth=Simplest  InputSameDT=off
  Relational Operator2 : RelationalOperator  OutDataTypeStr=boolean  RndMeth=Simplest  InputSameDT=off
  Repeating Sequence : simulink/Sources/Repeating Sequence  rep_seq_t=[0 0.00005 0.0001]  rep_seq_y=[-1 1 -1]
  PWM1 : Outport
  PWM2 : Outport  Port=2
  PWM3 : Outport  Port=3
  PWM4 : Outport  Port=4
  PWM5 : Outport  Port=5
  PWM6 : Outport  Port=6
  wires:
  Vbref/1 -> Relational Operator1/1
  Relational Operator1/1 -> PWM3/1, Logical Operator1/1
  Repeating Sequence/1 -> Relational Operator1/2, Relational Operator/2, Relational Operator2/2
  Relational Operator/1 -> PWM1/1, Logical Operator/1
  Vcref/1 -> Relational Operator2/1
  Logical Operator1/1 -> PWM4/1
  Logical Operator/1 -> PWM2/1
  Relational Operator2/1 -> PWM5/1, Logical Operator2/1
  Logical Operator2/1 -> PWM6/1
  Varef/1 -> Relational Operator/1

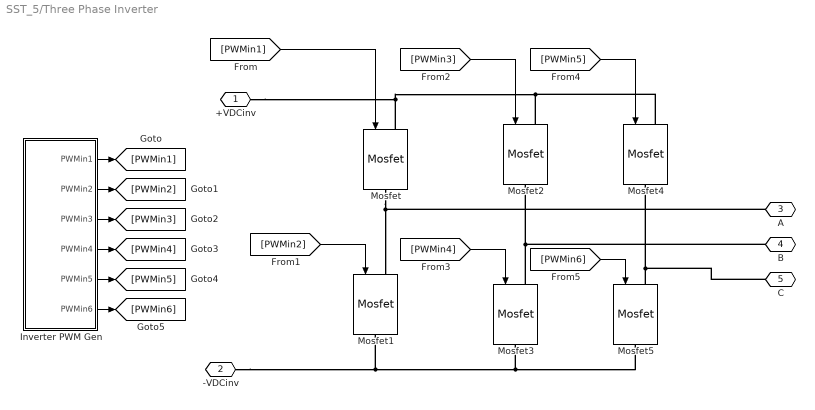
== system SST_5/Three Phase Inverter ==
  "Inverter PWM Gen " : Subsystem
  Mosfet{,1..5} (6 alike) : spsMosfetLib/Mosfet  Ron=0.1  Lon=0  Rd=0.01  Vfd=0  IC=0  Rs=1e5  Cs=inf  Measurements=off
  +VDCinv : PMIOPort  Side=Left
  -VDCinv : PMIOPort  Port=2  Side=Left
  A : PMIOPort  Port=3  Side=Right
  B : PMIOPort  Port=4  Side=Right
  C : PMIOPort  Port=5  Side=Right
  wires:
  [PWMin3] -> Mosfet2/1
  [PWMin5] -> Mosfet4/1
  [PWMin4] -> Mosfet3/1
  [PWMin1] -> Mosfet/1
  [PWMin2] -> Mosfet1/1
  [PWMin6] -> Mosfet5/1
  "Inverter PWM Gen "/3(PWMin3) -> [PWMin3]
  "Inverter PWM Gen "/5(PWMin5) -> [PWMin5]
  "Inverter PWM Gen "/2(PWMin2) -> [PWMin2]
  "Inverter PWM Gen "/1(PWMin1) -> [PWMin1]
  "Inverter PWM Gen "/6(PWMin6) -> [PWMin6]
  "Inverter PWM Gen "/4(PWMin4) -> [PWMin4]
  connections:
  B/RConn1 -- Mosfet3/LConn1 -- Mosfet2/RConn1
  +VDCinv/RConn1 -- Mosfet4/LConn1 -- Mosfet2/LConn1 -- Mosfet/LConn1
  A/RConn1 -- Mosfet/RConn1 -- Mosfet1/LConn1
  C/RConn1 -- Mosfet5/LConn1 -- Mosfet4/RConn1
  Mosfet1/RConn1 -- -VDCinv/RConn1 -- Mosfet5/RConn1 -- Mosfet3/RConn1

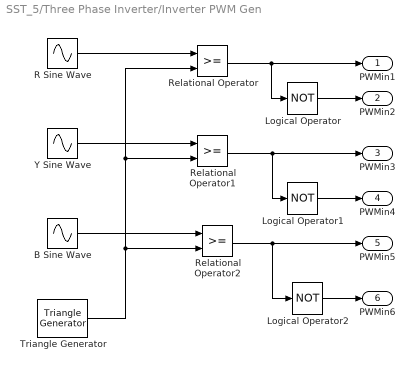
== system SST_5/Three Phase Inverter/Inverter PWM Gen  ==
  B Sine Wave : Sin  Amplitude=0.8  Frequency=2*pi*50  Phase=-2*pi*50/3  SampleTime=0
  Logical Operator : Logic  Operator=NOT  AllPortsSameDT=off  OutDataTypeStr=boolean
  Logical Operator1 : Logic  Operator=NOT  AllPortsSameDT=off  OutDataTypeStr=boolean
  Logical Operator2 : Logic  Operator=NOT  AllPortsSameDT=off  OutDataTypeStr=boolean
  R Sine Wave : Sin  Amplitude=0.8  Frequency=2*pi*50  SampleTime=0
  Relational Operator : RelationalOperator  OutDataTypeStr=boolean  RndMeth=Simplest  InputSameDT=off
  Relational Operator1 : RelationalOperator  OutDataTypeStr=boolean  RndMeth=Simplest  InputSameDT=off
  Relational Operator2 : RelationalOperator  OutDataTypeStr=boolean  RndMeth=Simplest  InputSameDT=off
  Triangle Generator : spsTriangleGeneratorLib/Triangle Generator  Freq=10e3  Phase=90  Ts=0
  Y Sine Wave : Sin  Amplitude=0.8  Frequency=2*pi*50  Phase=2*pi*50/3  SampleTime=0
  PWMin1 : Outport
  PWMin2 : Outport  Port=2
  PWMin3 : Outport  Port=3
  PWMin4 : Outport  Port=4
  PWMin5 : Outport  Port=5
  PWMin6 : Outport  Port=6
  wires:
  B Sine Wave/1 -> Relational Operator2/1
  Logical Operator/1 -> PWMin2/1
  Triangle Generator/1 -> Relational Operator2/2, Relational Operator1/2, Relational Operator/2
  Y Sine Wave/1 -> Relational Operator1/1
  Relational Operator/1 -> PWMin1/1, Logical Operator/1
  Relational Operator1/1 -> PWMin3/1, Logical Operator1/1
  Logical Operator1/1 -> PWMin4/1
  Logical Operator2/1 -> PWMin6/1
  Relational Operator2/1 -> PWMin5/1, Logical Operator2/1
  R Sine Wave/1 -> Relational Operator/1

== matlab function SST_5/DAB_with_IGBT/MATLAB Function ==
  data: time input; PWM2 output; frequency input; phase input; PWM1 output
function [PWM2, PWM1] = fcn(time, frequency, phase)

T_switching = 1/frequency;
PWM1 = 0;
PWM2 = 0;
x = mod(time, T_switching);
if x<T_switching/2
	PWM1 = 1;
end
t_phi = T_switching+phase/360;
y= mod(time+t_phi, T_switching);
if y<T_switching/2
	PWM2 = 1;
end
